simulink model "ABMS_FK_Optimization"  (R2024a)
settings: Solver=ode45  StartTime=0.0  StopTime=t1(end)  MaxStep=1e-4  RelTol=1e-3
model workspace (MAT data in the model file):
  SDO_OutputTimes = 0
values from neighbouring files (symbols this model uses):
  c_floor = 62.8188429312    [ForwardKinematicsReadyOptimization.mat]
  cAnkle = 1000    [ForwardKinematicsReadyOptimization.mat]
  cHat = 1000    [ForwardKinematicsReadyOptimization.mat]
  cHip = 1000    [ForwardKinematicsReadyOptimization.mat]
  cKnee = 1000    [ForwardKinematicsReadyOptimization.mat]
  d = 0.005    [ForwardKinematicsReadyOptimization.mat]
  dt = 0.00194789579158    [ForwardKinematicsReadyOptimization.mat]
  footCoG_x = 0.048032    [ForwardKinematicsReadyOptimization.mat]
  footCoG_y = 0.03081    [ForwardKinematicsReadyOptimization.mat]
  footHeight = 0.06162    [ForwardKinematicsReadyOptimization.mat]
  footInertia = 0.00070433888961    [ForwardKinematicsReadyOptimization.mat]
  footLength = 0.24016    [ForwardKinematicsReadyOptimization.mat]
  footMass = 0.82215    [ForwardKinematicsReadyOptimization.mat]
  hatCoG = -0.05733504    [ForwardKinematicsReadyOptimization.mat]
  hatInertia = 1.9582821044    [ForwardKinematicsReadyOptimization.mat]
  k_floor = 2646.94405241    [ForwardKinematicsReadyOptimization.mat]
  kAnkle = 11643.6295541    [ForwardKinematicsReadyOptimization.mat]
  kHat = 20655.7189422    [ForwardKinematicsReadyOptimization.mat]
  kHip = 10850.9172876    [ForwardKinematicsReadyOptimization.mat]
  kKnee = 36599.3663246    [ForwardKinematicsReadyOptimization.mat]
  L = 1.58    [ForwardKinematicsReadyOptimization.mat]
  M = 56.7    [ForwardKinematicsReadyOptimization.mat]
  omega_ankle_L = [-1.72946807619 -1.75737353503 -1.78034856033 -1.79855294145 -1.81216431593 -1.82137637434 -1.82639701034 -1.82744643093 -1.82475524177 -1.81856252257 -1.80911390714 -1.79665968238 ... (500 elements, 500x1)]    [ForwardKinematicsReadyOptimization.mat]
  omega_ankle_R = [2.03625246317 1.87895799946 1.71908308042 1.55696000935 1.39292869416 1.22733586468 1.06053424947 0.892881711684 0.724740343936 0.556475522401 0.388454920876 0.221047485982 ... (500 elements, 500x1)]    [ForwardKinematicsReadyOptimization.mat]
  omega_hip_L = [-0.280611688679 -0.311570063188 -0.345107260568 -0.38110500203 -0.419429739456 -0.459933358207 -0.502453986364 -0.546816904373 -0.592835548257 -0.640312598834 -0.68904114874 -0.738805938443 ... (500 elements, 500x1)]    [ForwardKinematicsReadyOptimization.mat]
  omega_hip_R = [2.436874577 2.50137810017 2.56518693791 2.62820305906 2.690326825 2.7514571145 2.81149146904 2.87032625968 2.92785687598 2.98397793742 3.03858352766 3.09156745152 ... (500 elements, 500x1)]    [ForwardKinematicsReadyOptimization.mat]
  omega_knee_L = [1.96123814792 1.91418307718 1.85419760709 1.78297919547 1.70210911406 1.61305682274 1.51718435711 1.41575071667 1.30991624212 1.20074697044 1.08921895698 0.976222554764 ... (500 elements, 500x1)]    [ForwardKinematicsReadyOptimization.mat]
  omega_knee_R = [-6.31491022355 -6.2996719536 -6.27749939257 -6.24831489493 -6.21206519479 -6.168721658 -6.11828036625 -6.06076203398 -5.99621176048 -5.92469862101 -5.84631510196 -5.76117638659 ... (500 elements, 500x1)]    [ForwardKinematicsReadyOptimization.mat]
  shankCoG = 0.02604156    [ForwardKinematicsReadyOptimization.mat]
  shankInertia = 0.0363273974795    [ForwardKinematicsReadyOptimization.mat]
  shankLength = 0.38868    [ForwardKinematicsReadyOptimization.mat]
  shankMass = 2.63655    [ForwardKinematicsReadyOptimization.mat]
  theta_ankle_L = [0.104089190059 0.10089407725 0.0976495615316 0.094363371469 0.0910429873004 0.0876956182925 0.0843281827148 0.0809472904543 0.0775592282756 0.0741699477128 0.070785055563 0.0674098069326 ... (500 elements, 500x1)]    [ForwardKinematicsReadyOptimization.mat]
  theta_ankle_R = [0.268664443161 0.271247145186 0.273677847781 0.275939163558 0.27801459569 0.279888613303 0.281546720628 0.282975519613 0.284162765692 0.28509741648 0.285769673205 0.286171014728 ... (500 elements, 500x1)]    [ForwardKinematicsReadyOptimization.mat]
  theta_hip_L = [0.203866490768 0.203326556251 0.202708469588 0.202008986109 0.201225063456 0.20035388195 0.199392863962 0.198339692183 0.197192326665 0.195949020524 0.194608334197 0.19316914817 ... (500 elements, 500x1)]    [ForwardKinematicsReadyOptimization.mat]
  theta_hip_R = [-0.0372016659367 -0.0333395086271 -0.0292594880672 -0.0249651189751 -0.0204604325022 -0.0157499604189 -0.0108387175733 -0.00573218271268 -0.000436277763004 0.00504265433304 0.010697873109 0.0165222652855 ... (500 elements, 500x1)]    [ForwardKinematicsReadyOptimization.mat]
  theta_knee_L = [-0.239993153363 -0.245883098322 -0.251093519717 -0.255698925452 -0.259765380933 -0.263351270801 -0.266508012215 -0.269280721542 -0.271708836309 -0.273826694261 -0.275664071344 -0.277246680395 ... (500 elements, 500x1)]    [ForwardKinematicsReadyOptimization.mat]
  theta_knee_R = [-0.820430486691 -0.832341256015 -0.844266598336 -0.856189608949 -0.868093439005 -0.879961330014 -0.891776648203 -0.903522918602 -0.915183858758 -0.926743411958 -0.938185779838 -0.949495454282 ... (500 elements, 500x1)]    [ForwardKinematicsReadyOptimization.mat]
  thighCoG = 0.0259357    [ForwardKinematicsReadyOptimization.mat]
  thighInertia = 0.0886409590374    [ForwardKinematicsReadyOptimization.mat]
  thighLength = 0.3871    [ForwardKinematicsReadyOptimization.mat]
  thighMass = 5.67    [ForwardKinematicsReadyOptimization.mat]
  x_hip = [-8.44173174878e-05 0.00319684354612 0.00644879199438 0.00967154739147 0.0128652983927 0.0160302986852 0.0191668628036 0.0222753620261 0.0253562203613 0.0284099106285 0.0314369506394 0.0344378994863 ... (500 elements, 500x1)]    [ForwardKinematicsReadyOptimization.mat]
  y_hip = [0.786844713626 0.786912596344 0.786989490296 0.787076184105 0.787173456036 0.787282069444 0.787402768296 0.787536272813 0.787683275238 0.787844435773 0.788020378698 0.788211688702 ... (500 elements, 500x1)]    [ForwardKinematicsReadyOptimization.mat]
undefined symbols (not defined in the file or in its folder): omega_hat, X, Y, y_heel, Z
libraries: nesl_utility x77, sm_lib x60
(part 3 of 3)

== matlab function ABMS_FK_Optimization/R. Leg/GRF/Normal Force Calculator2 ==
  data: k input; c_max input; u input; y output; udot input
function y = fcn(k, c_max, u, udot)

%k = 1.5e4;
%c_max = 1500;
h = 0.01;

d = abs(u);
ddot = abs(udot);

    if u <= 0
        F_k = k*d;
        if d < h
            F_c = c_max*abs(3*(d/h)^2-2*(d/h)^3)*ddot;
        else
            F_c = c_max*ddot;
        end 
    else
        F_k = 0;
        F_c = 0;
    end

y = F_k + F_c;

== matlab function ABMS_FK_Optimization/R. Leg/GRF/Normal Force Calculator3 ==
  data: k input; c_max input; u input; y output; udot input
function y = fcn(k, c_max, u, udot)

%k = 1.5e4;
%c_max = 1500;
h = 0.01;

d = abs(u);
ddot = abs(udot);

    if u <= 0
        F_k = k*d;
        if d < h
            F_c = c_max*abs(3*(d/h)^2-2*(d/h)^3)*ddot;
        else
            F_c = c_max*ddot;
        end 
    else
        F_k = 0;
        F_c = 0;
    end

y = F_k + F_c;

== matlab function ABMS_FK_Optimization/R. Leg/GRF/Normal Force Calculator4 ==
  data: k input; c_max input; u input; y output; udot input
function y = fcn(k, c_max, u, udot)

%k = 1.5e4;
%c_max = 1500;
h = 0.01;

d = abs(u);
ddot = abs(udot);

    if u <= 0
        F_k = k*d;
        if d < h
            F_c = c_max*abs(3*(d/h)^2-2*(d/h)^3)*ddot;
        else
            F_c = c_max*ddot;
        end 
    else
        F_k = 0;
        F_c = 0;
    end

y = F_k + F_c;

== matlab function ABMS_FK_Optimization/R. Leg/GRF/Friction Force Calculator ==
  data: u input; y output; F_N input
function y = fcn(u, F_N)

    mu_s = 0.8;
    mu_d = 0.2;
    
    if sign(u) == 0
        S = 1;
    else
        S = sign(u);
    end
    
    if u < 0.05
        mu = mu_s;
    else
        mu = mu_d;
    end
y = -mu*S*F_N;

== matlab function ABMS_FK_Optimization/R. Leg/GRF/Friction Force Calculator1 ==
  data: u input; y output; F_N input
function y = fcn(u, F_N)

    mu_s = 0.8;
    mu_d = 0.2;
    
    if sign(u) == 0
        S = 1;
    else
        S = sign(u);
    end
    
    if u < 0.05
        mu = mu_s;
    else
        mu = mu_d;
    end
y = -mu*S*F_N;

== matlab function ABMS_FK_Optimization/R. Leg/GRF/Friction Force Calculator2 ==
  data: u input; y output; F_N input
function y = fcn(u, F_N)

    mu_s = 0.8;
    mu_d = 0.2;
    
    if sign(u) == 0
        S = 1;
    else
        S = sign(u);
    end
    
    if u < 0.05
        mu = mu_s;
    else
        mu = mu_d;
    end
y = -mu*S*F_N;

== matlab function ABMS_FK_Optimization/R. Leg/GRF/Friction Force Calculator3 ==
  data: u input; y output; F_N input
function y = fcn(u, F_N)

    mu_s = 0.8;
    mu_d = 0.2;
    
    if sign(u) == 0
        S = 1;
    else
        S = sign(u);
    end
    
    if u < 0.05
        mu = mu_s;
    else
        mu = mu_d;
    end
y = -mu*S*F_N;

== matlab function ABMS_FK_Optimization/R. Leg/GRF/Friction Force Calculator4 ==
  data: u input; y output; F_N input
function y = fcn(u, F_N)

    mu_s = 0.8;
    mu_d = 0.2;
    
    if sign(u) == 0
        S = 1;
    else
        S = sign(u);
    end
    
    if u < 0.05
        mu = mu_s;
    else
        mu = mu_d;
    end
y = -mu*S*F_N;
